simulink model "fuzz"  (R2020a)
settings: Solver=ode4  StartTime=0.0  StopTime=10.0  FixedStep=0.01  RelTol=1e-3
libraries: fuzblock x1
settings Model: Creator=Adrian  LastModifiedBy=Adrian
settings SolverCC: AlgebraicLoopSolver=LineSearch
settings RTWCC: RTWVerbose=off

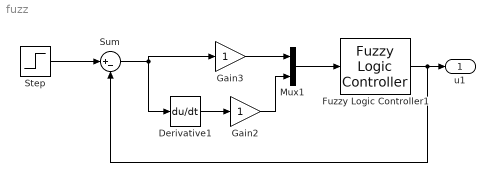
== system fuzz ==
  Derivative1 : Derivative
  Fuzzy Logic Controller1 : fuzblock/Fuzzy Logic  Controller  FIS='FUZZY_controller.fis'  OutputSampleNumber=101  DataType=double  FuzzifiedInputs=off  RuleFiringStrengths=off  RuleOutputs=off  AggregatedOutputs=off  SimulateUsing=Interpreted execution  OutOfRangeInputValueMessage=warning  NoRuleFiredMessage=warning  EmptyOutputFuzzySetMessage=warning
  Gain2 : Gain
  Gain3 : Gain
  Mux1 : Mux  Inputs=2
  Step : Step  Time=2  After=30  SampleTime=0
  Sum : Sum  Inputs=|+-
  u1 : Outport
  wires:
  Mux1/1 -> Fuzzy Logic Controller1/1
  Gain2/1 -> Mux1/2
  Gain3/1 -> Mux1/1
  Sum/1 -> Derivative1/1, Gain3/1
  Derivative1/1 -> Gain2/1
  Fuzzy Logic Controller1/1 -> Sum/2, u1/1
  Step/1 -> Sum/1
